simulink model "StaticVarCompensator"  (R2024a)
settings: Solver=FixedStepDiscrete  StartTime=0.0  StopTime=1  FixedStep=Ts  MaxStep=Ts*2  RelTol=1e-4  AbsTol=1e-4
PreLoadFcn:
  | Ts=50e-6;
undefined symbols (not defined in the file or in its folder): D1, Delta, DiscIntNeverNeededParam, find_system
libraries: spsSampleandHoldLib x24, spsThyristorLib x24, spsEdgeDetectorLib x12, spsSeriesRLCBranchLib x12, spsParallelRLCBranchLib x9, spsBistableLib x3, spsMeanVariableFrequencyLib x3, spsSecondOrderFilterLib x3, spsMultimeterLib x3, spsThreePhaseVIMeasurementLib x2, spsStairGeneratorLib x2, spsThreePhaseSeriesRLCLoadLib x1
(part 1 of 3)
settings Model: Creator=The MathWorks, Inc.  LastModifiedBy=Monia
settings SolverCC: AutoScaleAbsTol=off  AlgebraicLoopSolver=TrustRegion
settings DataIOCC: SaveFormat=StructureWithTime  SaveOutput=off  SignalLogging=off  DSMLogging=off  SaveTime=off  ReturnWorkspaceOutputs=off  SignalLoggingName=sigsOut
settings OptimizationCC: BooleanDataType=off  ExpressionDepthLimit=2147483647  InitFltsAndDblsToZero=on  EfficientMapNaN2IntZero=off  LifeSpan=inf
settings DebuggingCC: UnderspecifiedInitializationDetection=Classic  MergeDetectMultiDrivingBlocksExec=none  CheckExecutionContextPreStartOutputMsg=on  SignalResolutionControl=TryResolveAllWithWarning  MultiTaskDSMMsg=warning  MultiTaskCondExecSysMsg=none  FcnCallInpInsideContextMsg=warning  UnconnectedInputMsg=warning  UnconnectedOutputMsg=warning  UnconnectedLineMsg=warning  AllowSymbolicDim=off  StateNameClashWarn=warning  SFUnexpectedBacktrackingDiag=warning  SFNoUnconditionalDefaultTransitionDiag=warning  SFExecutionAtInitializationDiag=none  ArithmeticOperatorsInVariantConditions=warning
settings HardwareCC: ProdBitPerPointer=32  ProdBitPerSizeT=32  ProdBitPerPtrDiffT=32  ProdLargestAtomicFloat=None  ProdIntDivRoundTo=Undefined  ProdEndianess=Unspecified  ProdWordSize=32  ProdHWDeviceType=32-bit Generic  TargetUnknown=on
settings ModelReferenceCC: EnableRefExpFcnMdlSchedulingChecks=on  PropagateSignalLabelsOutOfModel=off
settings SFSimCC: SimUseLocalCustomCode=off  CustomCodeUndefinedFunction=UseInterfaceOnly
settings RTWCC: RTWUseLocalCustomCode=off  GPUComputeCapability=3.5  DLArmComputeVersion=19.05
settings CodeAppCC: StateflowObjectComments=on
settings GRTTargetCC: TargetLangStandard=C89/C90 (ANSI)  CombineOutputUpdateFcns=off  GRTInterface=on
settings ConfigComp: CovMetricSettings=dw  CovSaveCumulativeToWorkspaceVar=on  CovSaveSingleToWorkspaceVar=on  CovExternalEMLEnable=off  CovSFcnEnable=off
settings SimscapeCC: SimscapeNormalizeSystem=off

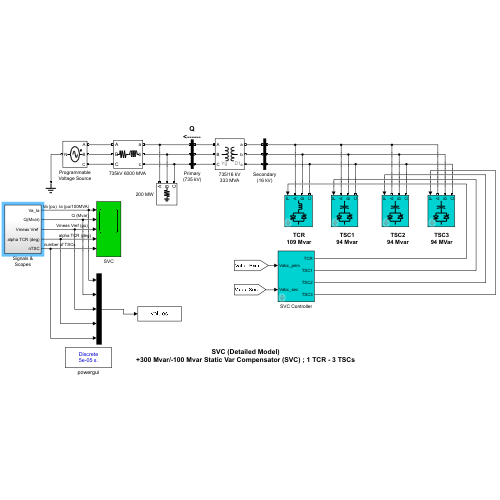
[thumbnail: Simulink's stored preview of the top-level diagram]
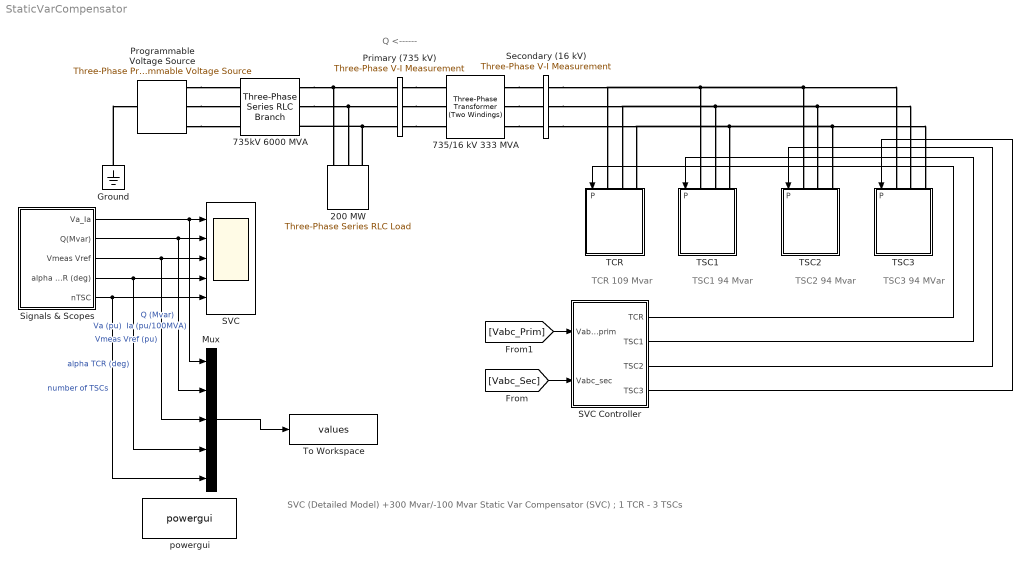
== system StaticVarCompensator ==
  note: SVC (Detailed Model)
      | +300 Mvar/-100 Mvar Static Var Compensator (SVC) ; 1 TCR - 3 TSCs
  note: TSC1
      | 94 Mvar
  note: TCR
      | 109 Mvar
  note: TSC2
      | 94 Mvar
  note: TSC3
      | 94 MVar
  note: Q
      | <------
  200 MW : spsThreePhaseSeriesRLCLoadLib/Three-Phase Series RLC Load  LConnTagsString=A|B|C  Configuration=Y (grounded)  NominalVoltage=735e3  Vabc=[1e3 1e3 1e3]  Vabcp=[1e3 1e3 1e3]  NominalFrequency=60  UnbalancedPower=off  ActivePower=200e6  InductivePower=0  CapacitivePower=0  Pabc=[10e3 9e3 11e3]  QLabc=[100 90 110]  QCabc=[100 90 110]  Pabcp=[10e3 9e3 11e3]  QLabcp=[100 90 110]  QCabcp=[100 90 110]  Measurements=None  LoadType=constant Z
  735/16 kV 333 MVA : spsThreePhaseTransformerTwoWindingsLib/Three-Phase Transformer (Two Windings)  Winding1Connection=Yg  Winding2Connection=Delta (D1)  CoreType=Three single-phase transformers  SetSaturation=off  Hysteresis=off  DataFile='hysteresis'  SetInitialFlux=off  Measurements=None  UNITS=pu  NominalPower=[333e6 , 60 ]  Winding1=[735e3 , 0.15/30/2 , 0.15*0.7]  Winding2=[ 16e3 , 0.15/30/2, 0.15*0.3]  Rm=500  Lm=500  L0=0.5  Saturation="[ 0,0  ;  0.005,1.2  ;  1.0,1.4 ]"  InitialFluxes=[ 0.8 , -0.8 , 0.7 ]  BreakLoop=off  DiscreteSolver=Trapezoidal iterative  DataType=off  TransfoNumber=0
  "735kV 6000 MVA " : spsThreePhaseSeriesRLCBranchLib/Three-Phase Series RLC Branch  LConnTagsString=A|B|C  RConnTagsString=A|B|C  BranchType=RL  Resistance=735e3^2/6000e6/10  Inductance=735e3^2/6000e6/(2*pi*60)  Capacitance=1.0  Measurements=None
  Ground : spsGroundLib/Ground  LConnTagsString=a
  Mux : Mux  Inputs=5
  Primary (735 kV) : spsThreePhaseVIMeasurementLib/Three-Phase V-I Measurement  VoltageMeasurement=phase-to-ground  SetLabelV=on  LabelV=Vabc_Prim  Vpu=on  VpuLL=off  CurrentMeasurement=yes  SetLabelI=on  LabelI=Iabc_Prim  Ipu=on  Pbase=100e6  Vbase=735e3  OutputType=Magnitude  PhasorSimulation=off  PSBequivalent=0
  Programmable Voltage Source : spsThreePhaseProgrammableVoltageSourceLib/Three-Phase Programmable Voltage Source  PositiveSequence="[1.004*735e3 0  60]"  VariationEntity=Amplitude  VariationType=Table of time-amplitude pairs  VariationTypeAlt=Step  VariationStep=-0.3  VariationRate=0.5  VariationMagnitude=0.4  VariationFrequency=2  VariationTiming=[0.1 1.2]  VariationPhaseA=off  Amplitudes=[1.0 1.025 0.93 1.0 ]  TimeValues=[0 0.1 0.4 0.7]  HarmonicGeneration=off  HarmonicA=[3 0.2 -25 0]  HarmonicB="[2 0.15  35 2]"  Timing="[0.1  0.6]"  BusType=swing  Pref=0  Qref=0  Qmin=-inf  Qmax=inf
  SVC : Scope  NumInputPorts=5
  SVC Controller : Subsystem  mask(SVC Controller){OpMode=Voltage regulation, Vref=1.0, KpKi=[0 800], Xs=0.01, Bmin_max=[-1.04  3.23], Bref=0, Ts=Ts}
      mask prompts: OpMode "Operation mode"; Vref "Reference voltage (pu):"; KpKi "Regulator gains [ Kp  Ki ]:"; Xs "Droop (pu/100MVA):"; Bmin_max "Min. and max. primary susceptances [ Bind Bcap] (pu/100MVA):"; Bref "Susceptance Bref (pu/100MVA) (Var control mode):"; Ts "Sample time (s):"
      mask help:
      | This block implements a controller for a Static Var Compensator (SVC) consisting of one thyristor-controlled reactor bank (TCR) and three thyristor-switched capacitor banks (TSCs). Outputs TCR, TSC1, TSC2 and TSC3 are vectors of six pulses for the TCR and the three TSCs.
      | In Voltage control mode the primary voltage (Vabc_prim) is controlled at Vref within the maximum inductive and capacitive susceptance range and droop setting. In Var control mode the SVC susceptance  is  kept constant at Bref (Bref<0 for inductive mode).
      | Thyristor pulses are synchronized on secondary line-to-line voltages (Vabc_sec) of the coupling transformer, assuming a Wye/Delta (D1) connection.
      mask init:
      | Kp=KpKi(1);
      | Ki=KpKi(2);
      | Bmin=Bmin_max(1);
      | Bmax=Bmin_max(2);
      mask TypeOptions OpMode: Voltage regulation | Var control (Fixed susceptance Bref)
  Secondary (16 kV) : spsThreePhaseVIMeasurementLib/Three-Phase V-I Measurement  VoltageMeasurement=phase-to-phase  SetLabelV=on  LabelV=Vabc_Sec  Vpu=on  VpuLL=off  CurrentMeasurement=no  SetLabelI=off  LabelI=Iabc_Sec  Ipu=off  Pbase=100e6  Vbase=16e3  OutputType=Magnitude  PhasorSimulation=off  PSBequivalent=0
  Signals & Scopes : Subsystem
  TCR : Subsystem  LoadFcn=find_system(gcs,'FollowLinks', 'on', 'LookUnderMasks', 'all');  mask(TCR branch){Ltcr=18.7e-3, Q=50, ParS=[500 250e-9], ParT=[1e-3  1*15]}
      mask prompts: Ltcr "TCR Inductance (H) :"; Q "Quality factor:"; ParS "Thyristor snubber: [ R (ohm)   C (F)  ]"; ParT "Thyristor data: [ Ron (ohm)   Vf (volt) ]"
      mask init:
      | Rtcr=(2*pi*60) * Ltcr / Q;
      | Rsnub=ParS(1);
      | Csnub=ParS(2);
      | Ron=ParT(1);
      | Vf=ParT(2);
      mask Display:
      | plot(0,0);plot(125,220)
      | plot([62 62 37 37 49 25 37],[15 39 39 58 76 76 58])
      | plot([62 87 87 99 87 75 87],[39 39 58 58 76 58 58])
      | plot([25 49],[58 58]);plot([37 25],[58 49])
      | plot([75 99],[76 76]);plot([87 99],[76 85])
      | plot([37 37 87 87],[76 95 95 76])
      | plot([62 62],[95 122]);plot([62 62],[164 186])
      | plot([62 72 78 79 78 72 62],[122 123 125 129 133 135 136])
      | plot([62 72 78 79 78 72 62],14+[122 123 125 129 133 135 136])
      | plot([62 72 78 79 78 72 62],28+[122 123 125 129 133 135 136])
  TSC1 : Subsystem  mask(TSC branch){Ccmt=308.4e-6, ParL=[1.13e-3 4.26e-3*2 191.7/2], ParS=[500 250e-9], ParT=[1e-3  1*15]}
      mask prompts: Ccmt "Capacitance (F) :"; ParL "[ Inductance (H)  Rseries (ohm)  Rparallel (ohm)  ]"; ParS "Thyristor snubber: [ R (ohm)   C (F)  ]"; ParT "Thyristor data: [ Ron (ohm)  Vf (volt) ]"
      mask init:
      | Lcmt=ParL(1);
      | Rseries=ParL(2);
      | Rparallel=ParL(3);
      | Rsnub=ParS(1);
      | Csnub=ParS(2);
      | Ron=ParT(1);
      | Vf=ParT(2);
      mask Display:
      | plot(0,0);plot(125,220)
      | plot([62 62 37 37 49 25 37],[15 39 39 58 76 76 58])
      | plot([62 87 87 99 87 75 87],[39 39 58 58 76 58 58])
      | plot([25 49],[58 58]);plot([37 25],[58 49])
      | plot([75 99],[76 76]);plot([87 99],[76 85])
      | plot([37 37 87 87],[76 95 95 76])
      | plot([62 62],[95 133]);plot([62 62],[164 183])
      | plot([62 69 73 78 81 82],13+[120 120 119 118 117 115])
      | plot([62 55 51 46 43 42],13+[120 120 119 118 117 115])
      | plot([42 82],[145 145])
      | plot([62 62],[145 164])
  TSC2 : Subsystem  mask(TSC branch){Ccmt=308.4e-6, ParL=[1.13e-3 4.26e-3*2 191.7/2], ParS=[500 250e-9], ParT=[1e-3 1*15]}
      mask prompts: Ccmt "Capacitance (F) :"; ParL "[ Inductance (H)  Rseries (ohm)  Rparallel (ohm)  ]"; ParS "Thyristor snubber: [ R (ohm)   C (F)  ]"; ParT "Thyristor data: [ Ron (ohm)  Vf (volt) ]"
      mask init:
      | Lcmt=ParL(1);
      | Rseries=ParL(2);
      | Rparallel=ParL(3);
      | Rsnub=ParS(1);
      | Csnub=ParS(2);
      | Ron=ParT(1);
      | Vf=ParT(2);
      mask Display:
      | plot(0,0);plot(125,220)
      | plot([62 62 37 37 49 25 37],[15 39 39 58 76 76 58])
      | plot([62 87 87 99 87 75 87],[39 39 58 58 76 58 58])
      | plot([25 49],[58 58]);plot([37 25],[58 49])
      | plot([75 99],[76 76]);plot([87 99],[76 85])
      | plot([37 37 87 87],[76 95 95 76])
      | plot([62 62],[95 133]);plot([62 62],[164 183])
      | plot([62 69 73 78 81 82],13+[120 120 119 118 117 115])
      | plot([62 55 51 46 43 42],13+[120 120 119 118 117 115])
      | plot([42 82],[145 145])
      | plot([62 62],[145 164])
  TSC3 : Subsystem  mask(TSC branch){Ccmt=308.4e-6, ParL=[1.13e-3 4.26e-3*2 191.7/2], ParS=[500 250e-9], ParT=[1e-3 1*15]}
      mask prompts: Ccmt "Capacitance (F) :"; ParL "[ Inductance (H)  Rseries (ohm)  Rparallel (ohm)  ]"; ParS "Thyristor snubber: [ R (ohm)   C (F)  ]"; ParT "Thyristor data: [ Ron (ohm)  Vf (volt) ]"
      mask init:
      | Lcmt=ParL(1);
      | Rseries=ParL(2);
      | Rparallel=ParL(3);
      | Rsnub=ParS(1);
      | Csnub=ParS(2);
      | Ron=ParT(1);
      | Vf=ParT(2);
      mask Display:
      | plot(0,0);plot(125,220)
      | plot([62 62 37 37 49 25 37],[15 39 39 58 76 76 58])
      | plot([62 87 87 99 87 75 87],[39 39 58 58 76 58 58])
      | plot([25 49],[58 58]);plot([37 25],[58 49])
      | plot([75 99],[76 76]);plot([87 99],[76 85])
      | plot([37 37 87 87],[76 95 95 76])
      | plot([62 62],[95 133]);plot([62 62],[164 183])
      | plot([62 69 73 78 81 82],13+[120 120 119 118 117 115])
      | plot([62 55 51 46 43 42],13+[120 120 119 118 117 115])
      | plot([42 82],[145 145])
      | plot([62 62],[145 164])
  To Workspace : ToWorkspace  VariableName=values  SaveFormat=Timeseries  SampleTime=-1
  powergui : spspowerguiLib/powergui  Priority=2  SimulationMode=Discrete  SampleTime=Ts  frequency=60  Iterations=50  frequencyindice=60  Pbase=100e6  ErrMax=1e-4  UnitsV=kV  UnitsW=MW  buscounter=0  FunctionMessages=off  echomessages=off  EnableUseOfTLC=off  CurrentSourceSwitches=off  DisableSnubberDevices=off  DisableRonSwitches=off  DisableVfSwitches=off  DisplayEquations=off  AutomaticDiscreteSolvers=off  SolverType=Tustin/Backward Euler (TBE)  Interpol=off  ExternalGateDelay=off  methode=off  Ts=0  x0status=blocks  SPID=off  SwTol=0  HookPort=off  NonlinearTolerance=0  nMaxIteration=15  ContinueOnMaxIteration=off  RestoreLinks=warning  ResistiveCurrentMeasurement=off  Frange=[0:2:500]  Ylog=off  Xlog=on  ShowGrid=off  save=off  variable=ZData  structure=0  ZoomFFT=on  StartTime=0.0  cycles=1  DisplayStyle=1  fundamental=60  FreqAxis=off  MaxFrequency=1000  frequencyindicesteady=1  RmsSteady=2  display=off
  wires:
  [Vabc_Sec] -> SVC Controller/2(Vabc_sec)
  [Vabc_Prim] -> SVC Controller/1(Vabc_prim)
  Signals & Scopes/1(Va_Ia) -> Mux/1, SVC/1  "Va (pu)  Ia (pu/100MVA)"
  SVC Controller/1(TCR) -> TCR/1(P)
  SVC Controller/2(TSC1) -> TSC1/1(P)
  SVC Controller/3(TSC2) -> TSC2/1(P)
  SVC Controller/4(TSC3) -> TSC3/1(P)
  Signals & Scopes/3("Vmeas Vref ") -> Mux/3, SVC/3  "Vmeas Vref (pu)"
  Signals & Scopes/5(nTSC) -> Mux/5, SVC/5  "number of TSCs"
  Signals & Scopes/2(Q(Mvar)) -> Mux/2, SVC/2  "Q (Mvar)"
  Signals & Scopes/4(alpha TCR (deg)) -> Mux/4, SVC/4  "alpha TCR (deg)"
  Mux/1 -> To Workspace/1
  connections:
  Ground/LConn1 -- Programmable Voltage Source/LConn1
  "735kV 6000 MVA "/RConn1 -- Primary (735 kV)/LConn1 -- 200 MW/LConn1
  "735kV 6000 MVA "/RConn2 -- Primary (735 kV)/LConn2 -- 200 MW/LConn2
  735/16 kV 333 MVA/RConn1 -- Secondary (16 kV)/LConn1
  735/16 kV 333 MVA/RConn3 -- Secondary (16 kV)/LConn3
  Programmable Voltage Source/RConn2 -- "735kV 6000 MVA "/LConn2
  Programmable Voltage Source/RConn3 -- "735kV 6000 MVA "/LConn3
  Programmable Voltage Source/RConn1 -- "735kV 6000 MVA "/LConn1
  735/16 kV 333 MVA/RConn2 -- Secondary (16 kV)/LConn2
  200 MW/LConn3 -- Primary (735 kV)/LConn3 -- "735kV 6000 MVA "/RConn3
  Secondary (16 kV)/RConn1 -- TCR/LConn1 -- TSC1/LConn1 -- TSC2/LConn1 -- TSC3/LConn1
  Secondary (16 kV)/RConn2 -- TCR/LConn2 -- TSC1/LConn2 -- TSC2/LConn2 -- TSC3/LConn2
  Secondary (16 kV)/RConn3 -- TCR/LConn3 -- TSC1/LConn3 -- TSC2/LConn3 -- TSC3/LConn3
  Primary (735 kV)/RConn1 -- 735/16 kV 333 MVA/LConn1
  Primary (735 kV)/RConn2 -- 735/16 kV 333 MVA/LConn2
  Primary (735 kV)/RConn3 -- 735/16 kV 333 MVA/LConn3

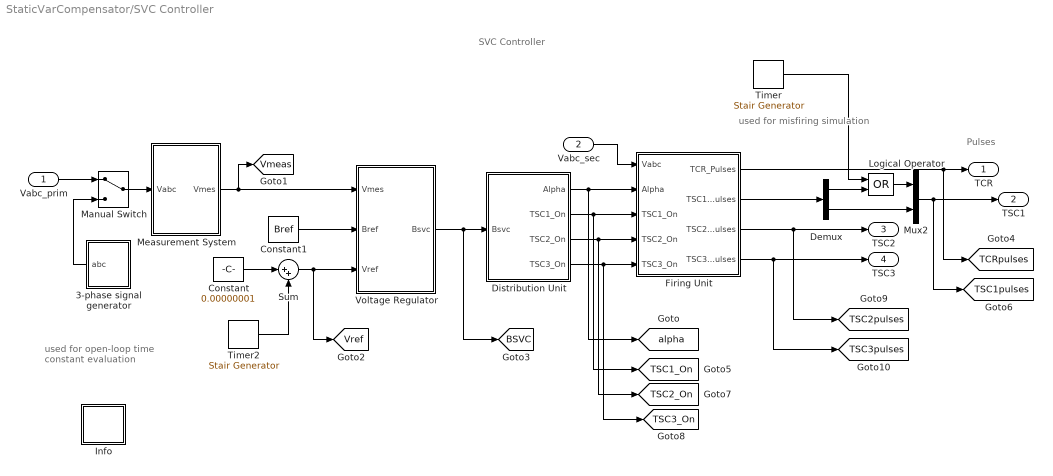
== system StaticVarCompensator/SVC Controller ==
  note: Pulses
  note: SVC Controller
  note: used for misfiring
      | simulation
  note: used for open-loop
      | time constant evaluation
  Vabc_prim : Inport  PortDimensions=3
  Vabc_sec : Inport  Port=2  PortDimensions=3
  3-phase signal generator : Subsystem
  Constant : Constant  Value=0.00000001
  Constant1 : Constant  Value=Bref
  Demux : Demux  Outputs=[1 5]
      settings: DisplayOption=none
  Distribution Unit : Subsystem  mask(Distribution Unit){ParNom=[333e6 60], Xf_xfo=0.15, Vsec_svc=16e3, L_TCR=18.7e-3, C_TSC=308.4e-6, L_TSC=1.13e-3, hyst_svc=0.1, Ts=Ts}
      mask prompts: ParNom "Transformer nominal power and frequency: [  P (VA)    Freq (Hz)  ]"; Xf_xfo "Transformer total leakage (pu/Pnom):"; Vsec_svc "Nominal secondary voltage (Volts rms ph-ph):"; L_TCR "TCR branch inductance (H):"; C_TSC "TSC branch capacitance (F):"; L_TSC "TSC branch inductance (H)"; hyst_svc "Hysteresis - Distribution unit (pu/100MVA):"; Ts "Sample time:"
      mask init:
      | Pnom_xfo=ParNom(1);
      | Freq=ParNom(2);
      | Bsec_pu100=100e6/Vsec_svc/Vsec_svc/3;
      | w=2*pi*Freq;
      | Bpu_TCR=-1/L_TCR/w/Bsec_pu100;
      | Bpu_TSC=1/(1/w/C_TSC-L_TSC*w)/Bsec_pu100;
      | B=1:-0.0025:0.0;
      | B=B';
      | for i=1:401,
      |       if B(i) <= 0,
      | 	ang = 0;
      |       elseif B(i) >= 1,
      | 	ang = pi;
      |       else,
      | 	a = pi; e = .0001;
      | 	da = a;
      | 	while abs(da)>e,
      | 		da = (pi*B(i)-a+sin(a))/(1-cos(a));
      | 		a = a + da;
      | 	end;
      | 	ang = a;
      |       end;
      |       A(i)=(180-ang*180/pi)/2+90;
      | end
      | A=A';
      | B=-B;
  Firing Unit : Subsystem  mask(Firing Unit){FiringMode=Synchronized, Nstep=0, ParInit=[0 60], Ts=Ts}
      mask prompts: FiringMode "Firing mode"; Nstep "Total delay (in number of time step)"; ParInit "Initial phase and frequency of input: [ Phase (degree)  Freq (Hz) ]"; Ts "Sample time:"
      mask init:
      | PhaseInit=ParInit(1);
      | FreqInit=ParInit(2);
      mask TypeOptions FiringMode: Synchronized | Continuous
  Info : Subsystem
      mask Display: disp('?')
  Logical Operator : Logic  Operator=OR
  Manual Switch : ManualSwitch
  Measurement System : Subsystem  mask(SVC measurement system){Vnom=735e3, ParI=[735e3*0.9998 0 60], Ts=Ts}
      mask prompts: Vnom "Nominal voltage (volts rms ph-ph)"; ParI "Initial input: [ Mag (volts rms ph-ph)  Phase (degree) Freq (Hz) ]"; Ts "Sample time:"
      mask init:
      | Mag_Init=ParI(1)/Vnom;
      | Phase_Init=ParI(2);
      | Freq_Init=ParI(3);
  Mux2 : Mux  Inputs=[1 5]
  Sum : Sum  Inputs=|++  SaturateOnIntegerOverflow=on
  Timer : spsStairGeneratorLib/Stair Generator  t="[ 0  0.121  0.121+eps ]*100"  e="[0  1  0 ]"  Ts=Ts
  Timer2 : spsStairGeneratorLib/Stair Generator  t="[ 0  0.4  0.6 ]"  e=[1 1 1 ]  Ts=Ts
  Voltage Regulator : Subsystem
  TCR : Outport  VectorParamsAs1DForOutWhenUnconnected=off
  TSC1 : Outport  Port=2  VectorParamsAs1DForOutWhenUnconnected=off
  TSC2 : Outport  Port=3  VectorParamsAs1DForOutWhenUnconnected=off
  TSC3 : Outport  Port=4  VectorParamsAs1DForOutWhenUnconnected=off
  tag scope: BSVC=global, TCRpulses=global, TSC1_On=global, TSC1pulses=global, TSC2_On=global, TSC2pulses=global, TSC3_On=global, TSC3pulses=global, Vmeas=global, Vref=global, alpha=global
  wires:
  Timer/1 -> Logical Operator/1
  Firing Unit/2(TSC1_Pulses) -> Demux/1
  Measurement System/1(Vmes) -> Voltage Regulator/1(Vmes), [Vmeas]
  Constant1/1 -> Voltage Regulator/2(Bref)
  Mux2/1 -> TSC1/1, [TSC1pulses]
  Demux/2 -> Mux2/2
  Logical Operator/1 -> Mux2/1
  Demux/1 -> Logical Operator/2
  Voltage Regulator/1(Bsvc) -> Distribution Unit/1(Bsvc), [BSVC]
  Sum/1 -> [Vref], Voltage Regulator/3(Vref)
  Constant/1 -> Sum/1
  Vabc_prim/1 -> Manual Switch/1
  Manual Switch/1 -> Measurement System/1(Vabc)
  3-phase signal generator/1(abc) -> Manual Switch/2
  Firing Unit/1(TCR_Pulses) -> TCR/1, [TCRpulses]
  Firing Unit/3(TSC2_Pulses) -> TSC2/1, [TSC2pulses]
  Firing Unit/4(TSC3_Pulses) -> TSC3/1, [TSC3pulses]
  Distribution Unit/1(Alpha) -> Firing Unit/2(Alpha), [alpha]
  Distribution Unit/2(TSC1_On) -> Firing Unit/3(TSC1_On), [TSC1_On]
  Distribution Unit/3(TSC2_On) -> Firing Unit/4(TSC2_On), [TSC2_On]
  Distribution Unit/4(TSC3_On) -> Firing Unit/5(TSC3_On), [TSC3_On]
  Vabc_sec/1 -> Firing Unit/1(Vabc)
  Timer2/1 -> Sum/2

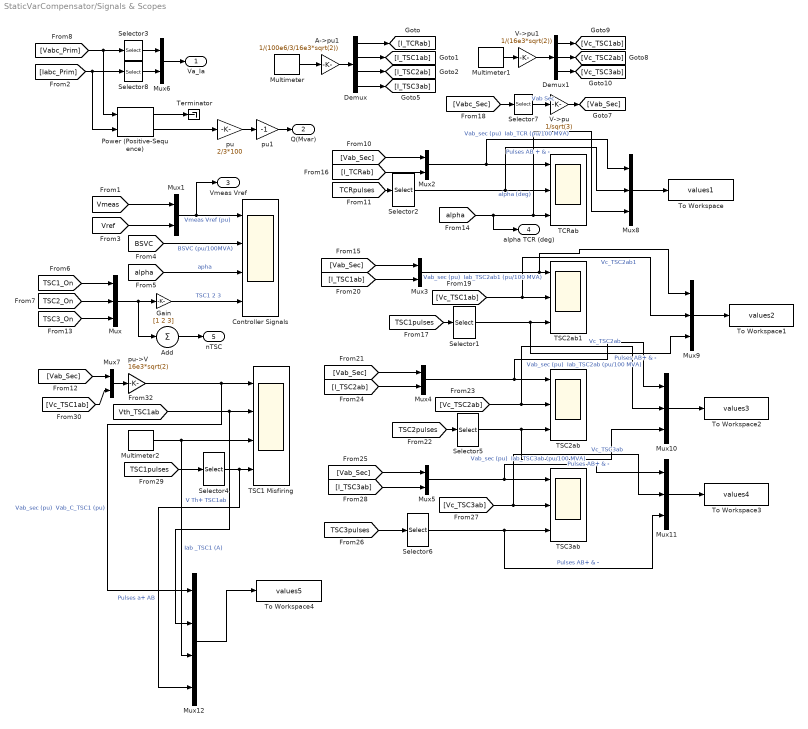
== system StaticVarCompensator/Signals & Scopes ==
  A->pu1 : Gain  Gain=1/(100e6/3/16e3*sqrt(2))  SaturateOnIntegerOverflow=on  OutDataTypeStr=Inherit: Same as input  ParamDataTypeStr=Inherit: Same as input
  Add : Sum  Inputs=+
  Controller Signals : Scope  NumInputPorts=4
  Demux : Demux
      settings: DisplayOption=none
  Demux1 : Demux  Outputs=3
      settings: DisplayOption=none
  Gain : Gain  Gain=[1 2 3]  SaturateOnIntegerOverflow=on  OutDataTypeStr=Inherit: Same as input  ParamDataTypeStr=Inherit: Same as input
  Multimeter : spsMultimeterLib/Multimeter  Tag=PoWeRsYsTeMmEaSuReMeNt  L=7  sel=[4 5 6 7]  yselected={}  Gain=[1 1 1 1]  OutputType=Magnitude  PlotAtSimulationStop=off  PhasorSimulation=off
      settings: AttributesFormatString=\n
  Multimeter1 : spsMultimeterLib/Multimeter  Tag=PoWeRsYsTeMmEaSuReMeNt  L=7  sel=[1 2 3]  yselected={}  Gain=[1 1 1]  OutputType=Magnitude  PlotAtSimulationStop=off  PhasorSimulation=off
      settings: AttributesFormatString=\n
  Multimeter2 : spsMultimeterLib/Multimeter  Tag=PoWeRsYsTeMmEaSuReMeNt  L=7  sel=5  yselected={}  Gain=1  OutputType=Magnitude  PlotAtSimulationStop=off  PhasorSimulation=off
      settings: AttributesFormatString=\n
  Mux{,8..11} (5 alike) : Mux  Inputs=3
  Mux{1..7} (7 alike) : Mux  Inputs=2
  Mux12 : Mux
  Power (Positive-Sequence) : spsPowerPositiveSequenceLib/Power (Positive-Sequence)  Freq=60  Vinit=[1 0]  Iinit=[0.05 90]  Ts=Ts
  Selector{1..2,5..6} (4 alike) : Selector  InputPortWidth=6  IndexOptions=Index vector (dialog)  Indices=[1 2]  OutputSizes=1
  Selector3 : Selector  InputPortWidth=3  IndexOptions=Index vector (dialog)  Indices=1  OutputSizes=1
  Selector4 : Selector  InputPortWidth=6  IndexOptions=Index vector (dialog)  Indices=[1 ]  OutputSizes=1
  Selector7 : Selector  InputPortWidth=3  IndexOptions=Index vector (dialog)  Indices=1  OutputSizes=1
  Selector8 : Selector  InputPortWidth=3  IndexOptions=Index vector (dialog)  Indices=1  OutputSizes=1
  TCRab : Scope  NumInputPorts=3
  TSC1 Misfiring : Scope  NumInputPorts=4
  TSC2ab : Scope  NumInputPorts=3
  TSC2ab1 : Scope  NumInputPorts=3
  TSC3ab : Scope  NumInputPorts=3
  Terminator : Terminator
  To Workspace : ToWorkspace  VariableName=values1  SaveFormat=Timeseries  SampleTime=-1
  To Workspace1 : ToWorkspace  VariableName=values2  SaveFormat=Timeseries  SampleTime=-1
  To Workspace2 : ToWorkspace  VariableName=values3  SaveFormat=Timeseries  SampleTime=-1
  To Workspace3 : ToWorkspace  VariableName=values4  SaveFormat=Timeseries  SampleTime=-1
  To Workspace4 : ToWorkspace  VariableName=values5  SaveFormat=Timeseries  SampleTime=-1
  "V->pu " : Gain  Gain=1/sqrt(3)  SaturateOnIntegerOverflow=on  OutDataTypeStr=Inherit: Same as input  ParamDataTypeStr=Inherit: Same as input
  V->pu1 : Gain  Gain=1/(16e3*sqrt(2))  SaturateOnIntegerOverflow=on  OutDataTypeStr=Inherit: Same as input  ParamDataTypeStr=Inherit: Same as input
  pu : Gain  Gain=2/3*100  SaturateOnIntegerOverflow=on  OutDataTypeStr=Inherit: Same as input  ParamDataTypeStr=Inherit: Same as input
  pu->V : Gain  Gain=16e3*sqrt(2)  SaturateOnIntegerOverflow=on  OutDataTypeStr=Inherit: Same as input  ParamDataTypeStr=Inherit: Same as input
  pu1 : Gain  Gain=-1  SaturateOnIntegerOverflow=on  OutDataTypeStr=Inherit: Same as input  ParamDataTypeStr=Inherit: Same as input
  Va_Ia : Outport  VectorParamsAs1DForOutWhenUnconnected=off
  Q(Mvar) : Outport  Port=2  VectorParamsAs1DForOutWhenUnconnected=off
  "Vmeas Vref " : Outport  Port=3  VectorParamsAs1DForOutWhenUnconnected=off
  alpha TCR (deg) : Outport  Port=4  VectorParamsAs1DForOutWhenUnconnected=off
  nTSC : Outport  Port=5  VectorParamsAs1DForOutWhenUnconnected=off
  wires:
  [TSC1_On] -> Mux/1
  [TSC2_On] -> Mux/2
  Mux/1 -> Gain/1, Add/1
  [Vmeas] -> Mux1/1
  [Vref] -> Mux1/2
  [Vabc_Prim] -> Power (Positive-Sequence)/1, Selector3/1
  [Iabc_Prim] -> Power (Positive-Sequence)/2, Selector8/1
  Power (Positive-Sequence)/1 -> Terminator/1
  pu/1 -> pu1/1
  [BSVC] -> Controller Signals/2  "BSVC (pu/100MVA)"
  Mux1/1 -> Controller Signals/1, "Vmeas Vref "/1  "Vmeas Vref (pu)"
  [alpha] -> Controller Signals/3  "apha"
  Gain/1 -> Controller Signals/4  "TSC1 2 3"
  [TSC3_On] -> Mux/3
  Multimeter/1 -> A->pu1/1
  [TCRpulses] -> Selector2/1
  Selector2/1 -> Mux8/2, TCRab/2  "Pulses AB + & -"
  Demux/1 -> [I_TCRab]
  Demux/4 -> [I_TSC3ab]
  [Vabc_Sec] -> Selector7/1
  Selector7/1 -> "V->pu "/1  "Vab Sec"
  [alpha] -> Mux8/3, TCRab/3, alpha TCR (deg)/1  "alpha (deg)"
  [Vab_Sec] -> Mux2/1
  [I_TCRab] -> Mux2/2
  Mux2/1 -> Mux8/1, TCRab/1  "Vab_sec (pu)  Iab_TCR (pu/100 MVA)"
  [Vab_Sec] -> Mux3/1
  [I_TSC1ab] -> Mux3/2
  [TSC1pulses] -> Selector1/1
  "V->pu "/1 -> [Vab_Sec]
  Demux/2 -> [I_TSC1ab]
  Demux/3 -> [I_TSC2ab]
  Multimeter1/1 -> V->pu1/1
  Demux1/1 -> [Vc_TSC1ab]
  Demux1/2 -> [Vc_TSC2ab]
  Demux1/3 -> [Vc_TSC3ab]
  [Vab_Sec] -> Mux4/1
  [I_TSC2ab] -> Mux4/2
  [TSC2pulses] -> Selector5/1
  [Vab_Sec] -> Mux5/1
  [I_TSC3ab] -> Mux5/2
  [TSC3pulses] -> Selector6/1
  pu1/1 -> Q(Mvar)/1
  Add/1 -> nTSC/1
  Selector3/1 -> Mux6/1
  Selector8/1 -> Mux6/2
  Mux6/1 -> Va_Ia/1
  [Vab_Sec] -> Mux7/1
  Mux7/1 -> pu->V/1
  [TSC1pulses] -> Selector4/1
  Selector4/1 -> Mux12/4, TSC1 Misfiring/4  "Pulses a+ AB"
  A->pu1/1 -> Demux/1
  V->pu1/1 -> Demux1/1
  [Vc_TSC1ab] -> Mux7/2
  Multimeter2/1 -> TSC1 Misfiring/3, Mux12/3  "Iab _TSC1 (A)"
  [Vth_TSC1ab] -> Mux12/2, TSC1 Misfiring/2  "V Th+ TSC1ab"
  pu->V/1 -> Mux12/1, TSC1 Misfiring/1  "Vab_sec (pu)  Vab_C_TSC1 (pu)"
  Power (Positive-Sequence)/2 -> pu/1
  Mux8/1 -> To Workspace/1
  Mux9/1 -> To Workspace1/1
  [Vc_TSC1ab] -> Mux9/2, TSC2ab1/2  "Vc_TSC2ab1"
  Mux3/1 -> Mux9/1, TSC2ab1/1  "Vab_sec (pu)  Iab_TSC2ab1 (pu/100 MVA)"
  Selector1/1 -> Mux9/3, TSC2ab1/3  "Pulses AB+ & -"
  Mux10/1 -> To Workspace2/1
  Mux4/1 -> Mux10/1, TSC2ab/1  "Vab_sec (pu)  Iab_TSC2ab (pu/100 MVA)"
  Selector5/1 -> Mux10/3, TSC2ab/3  "Pulses AB+ & -"
  [Vc_TSC2ab] -> Mux10/2, TSC2ab/2  "Vc_TSC2ab"
  Mux11/1 -> To Workspace3/1
  Mux5/1 -> Mux11/1, TSC3ab/1  "Vab_sec (pu)  Iab_TSC3ab (pu/100 MVA)"
  [Vc_TSC3ab] -> Mux11/2, TSC3ab/2  "Vc_TSC3ab"
  Selector6/1 -> Mux11/3, TSC3ab/3  "Pulses AB+ & -"
  Mux12/1 -> To Workspace4/1

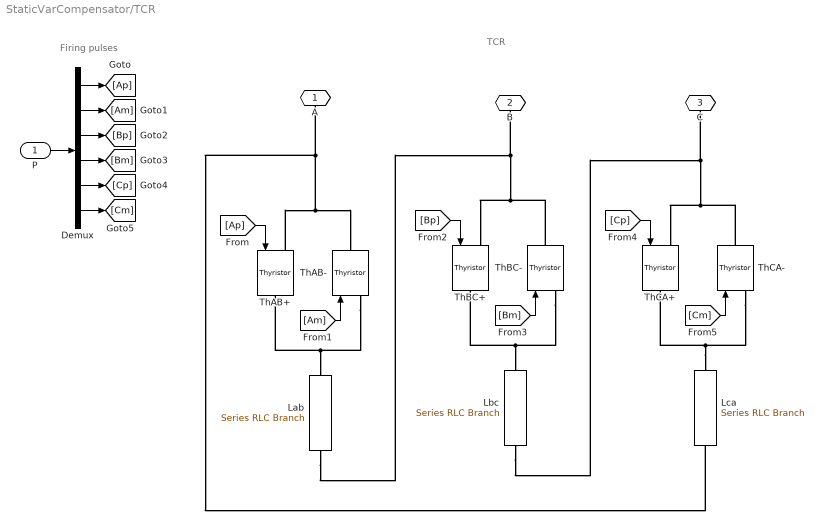
== system StaticVarCompensator/TCR ==
  note: Firing pulses
  note: TCR
  P : Inport  PortDimensions=6
  Demux : Demux  Outputs=6
      settings: DisplayOption=none
  Lab : spsSeriesRLCBranchLib/Series RLC Branch  LConnTagsString=__new0  RConnTagsString=__new0  BranchType=RL  Resistance=Rtcr  Inductance=Ltcr  SetiL0=off  InitialCurrent=0  Capacitance=1.0  Setx0=off  InitialVoltage=0  Measurements=Branch current
  Lbc : spsSeriesRLCBranchLib/Series RLC Branch  LConnTagsString=__new0  RConnTagsString=__new0  BranchType=RL  Resistance=Rtcr  Inductance=Ltcr  SetiL0=off  InitialCurrent=0  Capacitance=1.0  Setx0=off  InitialVoltage=0  Measurements=None
  Lca : spsSeriesRLCBranchLib/Series RLC Branch  LConnTagsString=__new0  RConnTagsString=__new0  BranchType=RL  Resistance=Rtcr  Inductance=Ltcr  SetiL0=off  InitialCurrent=0  Capacitance=1.0  Setx0=off  InitialVoltage=0  Measurements=None
  ThAB+ : spsThyristorLib/Thyristor  Ron=Ron  Lon=0  Vf=Vf  IC=0  Rs=Rsnub  Cs=Csnub  Measurements=off
      settings: AttributesFormatString=\n
  ThAB- : spsThyristorLib/Thyristor  Ron=Ron  Lon=0  Vf=Vf  IC=0  Rs=inf  Cs=0  Measurements=off
      settings: AttributesFormatString=\n
  ThBC+ : spsThyristorLib/Thyristor  Ron=Ron  Lon=0  Vf=Vf  IC=0  Rs=Rsnub  Cs=Csnub  Measurements=off
      settings: AttributesFormatString=\n
  ThBC- : spsThyristorLib/Thyristor  Ron=Ron  Lon=0  Vf=Vf  IC=0  Rs=inf  Cs=0  Measurements=off
      settings: AttributesFormatString=\n
  ThCA+ : spsThyristorLib/Thyristor  Ron=Ron  Lon=0  Vf=Vf  IC=0  Rs=Rsnub  Cs=Csnub  Measurements=off
      settings: AttributesFormatString=\n
  ThCA- : spsThyristorLib/Thyristor  Ron=Ron  Lon=0  Vf=Vf  IC=0  Rs=inf  Cs=0  Measurements=off
      settings: AttributesFormatString=\n
  A : PMIOPort  Side=Left
  B : PMIOPort  Port=2  Side=Left
  C : PMIOPort  Port=3  Side=Left
  wires:
  P/1 -> Demux/1
  Demux/1 -> [Ap]
  Demux/2 -> [Am]
  Demux/3 -> [Bp]
  Demux/4 -> [Bm]
  Demux/5 -> [Cp]
  [Cp] -> ThCA+/1
  [Cm] -> ThCA-/1
  Demux/6 -> [Cm]
  [Bm] -> ThBC-/1
  [Bp] -> ThBC+/1
  [Am] -> ThAB-/1
  [Ap] -> ThAB+/1
  connections:
  ThAB-/LConn1 -- ThAB+/RConn1 -- Lab/LConn1
  ThAB+/LConn1 -- ThAB-/RConn1 -- Lca/RConn1 -- A/RConn1
  ThBC-/LConn1 -- Lbc/LConn1 -- ThBC+/RConn1
  Lab/RConn1 -- ThBC-/RConn1 -- ThBC+/LConn1 -- B/RConn1
  Lca/LConn1 -- ThCA-/LConn1 -- ThCA+/RConn1
  Lbc/RConn1 -- ThCA-/RConn1 -- ThCA+/LConn1 -- C/RConn1

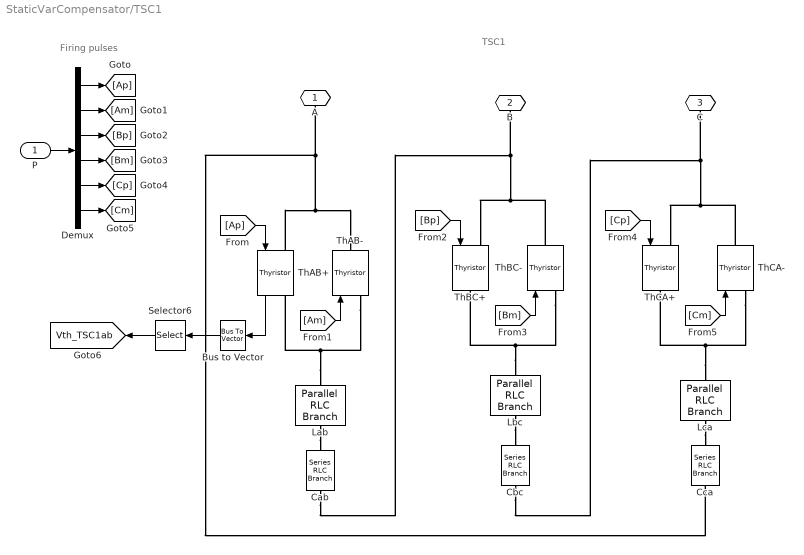
== system StaticVarCompensator/TSC1 ==
  note: Firing pulses
  note: TSC1
  P : Inport  PortDimensions=6
  Bus to Vector : BusToVector
  Cab : spsSeriesRLCBranchLib/Series RLC Branch  LConnTagsString=__new0  RConnTagsString=__new0  BranchType=RC  Resistance=Rseries  Inductance=1.0  SetiL0=off  InitialCurrent=0  Capacitance=Ccmt  Setx0=off  InitialVoltage=0  Measurements=Branch voltage and current
  Cbc : spsSeriesRLCBranchLib/Series RLC Branch  LConnTagsString=__new0  RConnTagsString=__new0  BranchType=RC  Resistance=Rseries  Inductance=1.0  SetiL0=off  InitialCurrent=0  Capacitance=Ccmt  Setx0=off  InitialVoltage=0  Measurements=None
  Cca : spsSeriesRLCBranchLib/Series RLC Branch  LConnTagsString=__new0  RConnTagsString=__new0  BranchType=RC  Resistance=Rseries  Inductance=1.0  SetiL0=off  InitialCurrent=0  Capacitance=Ccmt  Setx0=off  InitialVoltage=0  Measurements=None
  Demux : Demux  Outputs=6
      settings: DisplayOption=none
  Lab : spsParallelRLCBranchLib/Parallel RLC Branch  LConnTagsString=a  RConnTagsString=__new0  BranchType=RL  Resistance=Rparallel  Inductance=Lcmt  SetiL0=off  InitialCurrent=0  Capacitance=1.0  Setx0=off  InitialVoltage=0  Measurements=None
  Lbc : spsParallelRLCBranchLib/Parallel RLC Branch  LConnTagsString=a  RConnTagsString=__new0  BranchType=RL  Resistance=Rparallel  Inductance=Lcmt  SetiL0=off  InitialCurrent=0  Capacitance=1.0  Setx0=off  InitialVoltage=0  Measurements=None
  Lca : spsParallelRLCBranchLib/Parallel RLC Branch  LConnTagsString=a  RConnTagsString=__new0  BranchType=RL  Resistance=Rparallel  Inductance=Lcmt  SetiL0=off  InitialCurrent=0  Capacitance=1.0  Setx0=off  InitialVoltage=0  Measurements=None
  Selector6 : Selector  InputPortWidth=2  IndexOptions=Index vector (dialog)  Indices=2  OutputSizes=1
  ThAB+ : spsThyristorLib/Thyristor  Ron=Ron  Lon=0  Vf=Vf  IC=0  Rs=Rsnub  Cs=Csnub  Measurements=on
      settings: AttributesFormatString=\n
  ThAB- : spsThyristorLib/Thyristor  Ron=Ron  Lon=0  Vf=Vf  IC=0  Rs=inf  Cs=0  Measurements=off
      settings: AttributesFormatString=\n
  ThBC+ : spsThyristorLib/Thyristor  Ron=Ron  Lon=0  Vf=Vf  IC=0  Rs=Rsnub  Cs=Csnub  Measurements=off
      settings: AttributesFormatString=\n
  ThBC- : spsThyristorLib/Thyristor  Ron=Ron  Lon=0  Vf=Vf  IC=0  Rs=inf  Cs=0  Measurements=off
      settings: AttributesFormatString=\n
  ThCA+ : spsThyristorLib/Thyristor  Ron=Ron  Lon=0  Vf=Vf  IC=0  Rs=Rsnub  Cs=Csnub  Measurements=off
      settings: AttributesFormatString=\n
  ThCA- : spsThyristorLib/Thyristor  Ron=Ron  Lon=0  Vf=Vf  IC=0  Rs=inf  Cs=0  Measurements=off
      settings: AttributesFormatString=\n
  A : PMIOPort  Side=Left
  B : PMIOPort  Port=2  Side=Left
  C : PMIOPort  Port=3  Side=Left
  tag scope: Vth_TSC1ab=global
  wires:
  P/1 -> Demux/1
  [Ap] -> ThAB+/1
  Demux/1 -> [Ap]
  Demux/2 -> [Am]
  Demux/3 -> [Bp]
  Demux/4 -> [Bm]
  Demux/5 -> [Cp]
  [Am] -> ThAB-/1
  [Bp] -> ThBC+/1
  [Bm] -> ThBC-/1
  [Cp] -> ThCA+/1
  [Cm] -> ThCA-/1
  Demux/6 -> [Cm]
  ThAB+/1 -> Bus to Vector/1
  Selector6/1 -> [Vth_TSC1ab]
  Bus to Vector/1 -> Selector6/1
  connections:
  Lab/RConn1 -- Cab/LConn1
  Lab/LConn1 -- ThAB-/LConn1 -- ThAB+/RConn1
  Cca/RConn1 -- A/RConn1 -- ThAB+/LConn1 -- ThAB-/RConn1
  Lbc/LConn1 -- ThBC-/LConn1 -- ThBC+/RConn1
  Cab/RConn1 -- ThBC-/RConn1 -- ThBC+/LConn1 -- B/RConn1
  Lca/LConn1 -- ThCA-/LConn1 -- ThCA+/RConn1
  Cbc/RConn1 -- ThCA-/RConn1 -- ThCA+/LConn1 -- C/RConn1
  Lbc/RConn1 -- Cbc/LConn1
  Lca/RConn1 -- Cca/LConn1

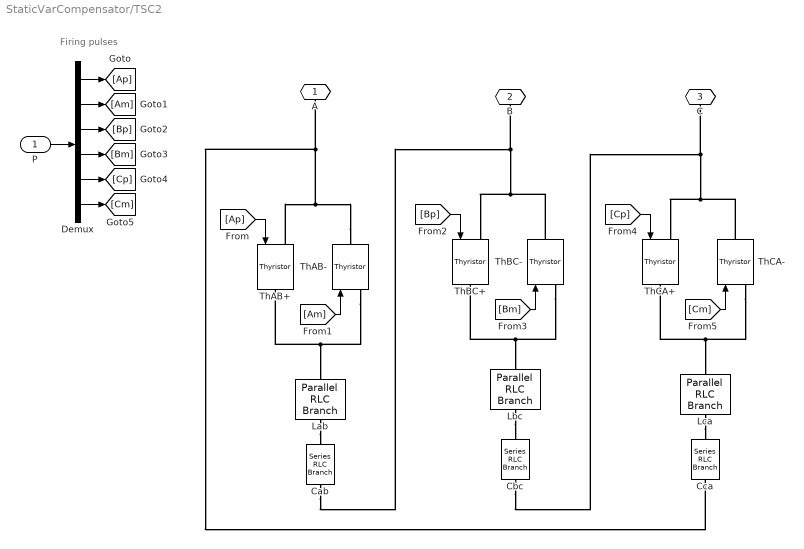
== system StaticVarCompensator/TSC2 ==
  note: Firing pulses
  P : Inport  PortDimensions=6
  Cab : spsSeriesRLCBranchLib/Series RLC Branch  LConnTagsString=__new0  RConnTagsString=__new0  BranchType=RC  Resistance=Rseries  Inductance=1.0  SetiL0=off  InitialCurrent=0  Capacitance=Ccmt  Setx0=off  InitialVoltage=0  Measurements=Branch voltage and current
  Cbc : spsSeriesRLCBranchLib/Series RLC Branch  LConnTagsString=__new0  RConnTagsString=__new0  BranchType=RC  Resistance=Rseries  Inductance=1.0  SetiL0=off  InitialCurrent=0  Capacitance=Ccmt  Setx0=off  InitialVoltage=0  Measurements=None
  Cca : spsSeriesRLCBranchLib/Series RLC Branch  LConnTagsString=__new0  RConnTagsString=__new0  BranchType=RC  Resistance=Rseries  Inductance=1.0  SetiL0=off  InitialCurrent=0  Capacitance=Ccmt  Setx0=off  InitialVoltage=0  Measurements=None
  Demux : Demux  Outputs=6
      settings: DisplayOption=none
  Lab : spsParallelRLCBranchLib/Parallel RLC Branch  LConnTagsString=a  RConnTagsString=__new0  BranchType=RL  Resistance=Rparallel  Inductance=Lcmt  SetiL0=off  InitialCurrent=0  Capacitance=1.0  Setx0=off  InitialVoltage=0  Measurements=None
  Lbc : spsParallelRLCBranchLib/Parallel RLC Branch  LConnTagsString=a  RConnTagsString=__new0  BranchType=RL  Resistance=Rparallel  Inductance=Lcmt  SetiL0=off  InitialCurrent=0  Capacitance=1.0  Setx0=off  InitialVoltage=0  Measurements=None
  Lca : spsParallelRLCBranchLib/Parallel RLC Branch  LConnTagsString=a  RConnTagsString=__new0  BranchType=RL  Resistance=Rparallel  Inductance=Lcmt  SetiL0=off  InitialCurrent=0  Capacitance=1.0  Setx0=off  InitialVoltage=0  Measurements=None
  ThAB+ : spsThyristorLib/Thyristor  Ron=Ron  Lon=0  Vf=Vf  IC=0  Rs=Rsnub  Cs=Csnub  Measurements=off
      settings: AttributesFormatString=\n
  ThAB- : spsThyristorLib/Thyristor  Ron=Ron  Lon=0  Vf=Vf  IC=0  Rs=inf  Cs=0  Measurements=off
      settings: AttributesFormatString=\n
  ThBC+ : spsThyristorLib/Thyristor  Ron=Ron  Lon=0  Vf=Vf  IC=0  Rs=Rsnub  Cs=Csnub  Measurements=off
      settings: AttributesFormatString=\n
  ThBC- : spsThyristorLib/Thyristor  Ron=Ron  Lon=0  Vf=Vf  IC=0  Rs=inf  Cs=0  Measurements=off
      settings: AttributesFormatString=\n
  ThCA+ : spsThyristorLib/Thyristor  Ron=Ron  Lon=0  Vf=Vf  IC=0  Rs=Rsnub  Cs=Csnub  Measurements=off
      settings: AttributesFormatString=\n
  ThCA- : spsThyristorLib/Thyristor  Ron=Ron  Lon=0  Vf=Vf  IC=0  Rs=inf  Cs=0  Measurements=off
      settings: AttributesFormatString=\n
  A : PMIOPort  Side=Left
  B : PMIOPort  Port=2  Side=Left
  C : PMIOPort  Port=3  Side=Left
  wires:
  Demux/6 -> [Cm]
  [Cm] -> ThCA-/1
  [Cp] -> ThCA+/1
  [Bm] -> ThBC-/1
  [Bp] -> ThBC+/1
  [Am] -> ThAB-/1
  Demux/5 -> [Cp]
  Demux/4 -> [Bm]
  Demux/3 -> [Bp]
  Demux/2 -> [Am]
  Demux/1 -> [Ap]
  [Ap] -> ThAB+/1
  P/1 -> Demux/1
  connections:
  Lca/RConn1 -- Cca/LConn1
  Lbc/RConn1 -- Cbc/LConn1
  C/RConn1 -- ThCA+/LConn1 -- ThCA-/RConn1 -- Cbc/RConn1
  ThCA+/RConn1 -- ThCA-/LConn1 -- Lca/LConn1
  B/RConn1 -- ThBC+/LConn1 -- ThBC-/RConn1 -- Cab/RConn1
  ThBC+/RConn1 -- ThBC-/LConn1 -- Lbc/LConn1
  ThAB-/RConn1 -- ThAB+/LConn1 -- A/RConn1 -- Cca/RConn1
  ThAB+/RConn1 -- ThAB-/LConn1 -- Lab/LConn1
  Lab/RConn1 -- Cab/LConn1

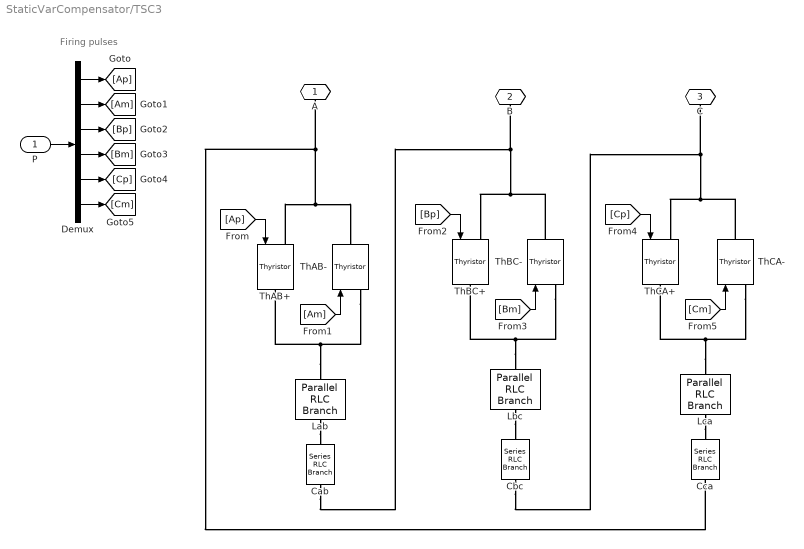
== system StaticVarCompensator/TSC3 ==
  note: Firing pulses
  P : Inport  PortDimensions=6
  Cab : spsSeriesRLCBranchLib/Series RLC Branch  LConnTagsString=__new0  RConnTagsString=__new0  BranchType=RC  Resistance=Rseries  Inductance=1.0  SetiL0=off  InitialCurrent=0  Capacitance=Ccmt  Setx0=off  InitialVoltage=0  Measurements=Branch voltage and current
  Cbc : spsSeriesRLCBranchLib/Series RLC Branch  LConnTagsString=__new0  RConnTagsString=__new0  BranchType=RC  Resistance=Rseries  Inductance=1.0  SetiL0=off  InitialCurrent=0  Capacitance=Ccmt  Setx0=off  InitialVoltage=0  Measurements=None
  Cca : spsSeriesRLCBranchLib/Series RLC Branch  LConnTagsString=__new0  RConnTagsString=__new0  BranchType=RC  Resistance=Rseries  Inductance=1.0  SetiL0=off  InitialCurrent=0  Capacitance=Ccmt  Setx0=off  InitialVoltage=0  Measurements=None
  Demux : Demux  Outputs=6
      settings: DisplayOption=none
  Lab : spsParallelRLCBranchLib/Parallel RLC Branch  LConnTagsString=a  RConnTagsString=__new0  BranchType=RL  Resistance=Rparallel  Inductance=Lcmt  SetiL0=off  InitialCurrent=0  Capacitance=1.0  Setx0=off  InitialVoltage=0  Measurements=None
  Lbc : spsParallelRLCBranchLib/Parallel RLC Branch  LConnTagsString=a  RConnTagsString=__new0  BranchType=RL  Resistance=Rparallel  Inductance=Lcmt  SetiL0=off  InitialCurrent=0  Capacitance=1.0  Setx0=off  InitialVoltage=0  Measurements=None
  Lca : spsParallelRLCBranchLib/Parallel RLC Branch  LConnTagsString=a  RConnTagsString=__new0  BranchType=RL  Resistance=Rparallel  Inductance=Lcmt  SetiL0=off  InitialCurrent=0  Capacitance=1.0  Setx0=off  InitialVoltage=0  Measurements=None
  ThAB+ : spsThyristorLib/Thyristor  Ron=Ron  Lon=0  Vf=Vf  IC=0  Rs=Rsnub  Cs=Csnub  Measurements=off
      settings: AttributesFormatString=\n
  ThAB- : spsThyristorLib/Thyristor  Ron=Ron  Lon=0  Vf=Vf  IC=0  Rs=inf  Cs=0  Measurements=off
      settings: AttributesFormatString=\n
  ThBC+ : spsThyristorLib/Thyristor  Ron=Ron  Lon=0  Vf=Vf  IC=0  Rs=Rsnub  Cs=Csnub  Measurements=off
      settings: AttributesFormatString=\n
  ThBC- : spsThyristorLib/Thyristor  Ron=Ron  Lon=0  Vf=Vf  IC=0  Rs=inf  Cs=0  Measurements=off
      settings: AttributesFormatString=\n
  ThCA+ : spsThyristorLib/Thyristor  Ron=Ron  Lon=0  Vf=Vf  IC=0  Rs=Rsnub  Cs=Csnub  Measurements=off
      settings: AttributesFormatString=\n
  ThCA- : spsThyristorLib/Thyristor  Ron=Ron  Lon=0  Vf=Vf  IC=0  Rs=inf  Cs=0  Measurements=off
      settings: AttributesFormatString=\n
  A : PMIOPort  Side=Left
  B : PMIOPort  Port=2  Side=Left
  C : PMIOPort  Port=3  Side=Left
  wires:
  P/1 -> Demux/1
  [Ap] -> ThAB+/1
  Demux/1 -> [Ap]
  Demux/2 -> [Am]
  Demux/3 -> [Bp]
  Demux/4 -> [Bm]
  Demux/5 -> [Cp]
  [Am] -> ThAB-/1
  [Bp] -> ThBC+/1
  [Bm] -> ThBC-/1
  [Cp] -> ThCA+/1
  [Cm] -> ThCA-/1
  Demux/6 -> [Cm]
  connections:
  Lab/RConn1 -- Cab/LConn1
  Lab/LConn1 -- ThAB-/LConn1 -- ThAB+/RConn1
  Cca/RConn1 -- A/RConn1 -- ThAB+/LConn1 -- ThAB-/RConn1
  Lbc/LConn1 -- ThBC-/LConn1 -- ThBC+/RConn1
  Cab/RConn1 -- ThBC-/RConn1 -- ThBC+/LConn1 -- B/RConn1
  Lca/LConn1 -- ThCA-/LConn1 -- ThCA+/RConn1
  Cbc/RConn1 -- ThCA-/RConn1 -- ThCA+/LConn1 -- C/RConn1
  Lbc/RConn1 -- Cbc/LConn1
  Lca/RConn1 -- Cca/LConn1

== system StaticVarCompensator/SVC Controller/3-phase signal generator ==
  Constant1 : Constant  Value=60
  Constant2 : Constant  Value=0.9998
  Constant3 : Constant  Value=-2
  Terminator : Terminator
  Three-Phase Sine Generator : spsThreePhaseSineGeneratorLib/Three-Phase Sine Generator  Ts=Ts
  abc : Outport  VectorParamsAs1DForOutWhenUnconnected=off
  wires:
  Constant1/1 -> Three-Phase Sine Generator/3
  Constant2/1 -> Three-Phase Sine Generator/1
  Constant3/1 -> Three-Phase Sine Generator/2
  Three-Phase Sine Generator/1 -> abc/1
  Three-Phase Sine Generator/2 -> Terminator/1

== system StaticVarCompensator/SVC Controller/Distribution Unit ==
  note: Bsec = ( 2 - Alpha/90 + sin(2*Alpha)/PI ) * Bsec_nom
  Bsvc : Inport  PortDimensions=1
  Bprim-->Bsec : Fcn  Expr=u[1]/(1 + u[1]*Xf_xfo*100e6/Pnom_xfo)
  Bsec --> Alpha : Lookup_n-D  NumberOfTableDimensions=1  BreakpointsForDimension1=B  BreakpointsForDimension2=[0 571.55 685.8 800.15 914.4 1028.8 1143.1 1257.4 1371.7 1486 1600.3 1714.6 1828.9 1943.2 2057.5 2171.8 2286.1 2400.5 2514.7 2629.1 2743.3 2857.7 2971.9 3086.3 3200.5 3314.9 3429.2]  Table=A  InternalRulePriority=Speed  RndMeth=Simplest
  Saturation : Saturate  UpperLimit=0  LowerLimit=Bpu_TCR
  Sum1 : Sum  Inputs=+---  InputSameDT=on  SaturateOnIntegerOverflow=on  OutDataTypeStr=Inherit: Same as first input
  TSC1 : Relay  OnSwitchValue=0  OffSwitchValue=-1 * hyst_svc
  TSC1+TSC2 : Relay  OnSwitchValue=0+ Bpu_TSC  OffSwitchValue=-1 * hyst_svc + Bpu_TSC
  TSC1+TSC2+TSC3 : Relay  OnSwitchValue=0+ 2*Bpu_TSC  OffSwitchValue=-1 * hyst_svc + 2*Bpu_TSC
  pu100_puLnom : Gain  Gain=-1/Bpu_TCR  SaturateOnIntegerOverflow=on  OutDataTypeStr=Inherit: Same as input  ParamDataTypeStr=Inherit: Same as input
  pu100_puLnom1 : Gain  Gain=Bpu_TSC  SaturateOnIntegerOverflow=on  OutDataTypeStr=Inherit: Same as input  ParamDataTypeStr=Inherit: Same as input
  pu100_puLnom2 : Gain  Gain=Bpu_TSC  SaturateOnIntegerOverflow=on  OutDataTypeStr=Inherit: Same as input  ParamDataTypeStr=Inherit: Same as input
  pu100_puLnom3 : Gain  Gain=Bpu_TSC  SaturateOnIntegerOverflow=on  OutDataTypeStr=Inherit: Same as input  ParamDataTypeStr=Inherit: Same as input
  Alpha : Outport  InitialOutput=0  VectorParamsAs1DForOutWhenUnconnected=off
  TSC1_On : Outport  Port=2  InitialOutput=0  VectorParamsAs1DForOutWhenUnconnected=off
  TSC2_On : Outport  Port=3  InitialOutput=0  VectorParamsAs1DForOutWhenUnconnected=off
  TSC3_On : Outport  Port=4  InitialOutput=0  VectorParamsAs1DForOutWhenUnconnected=off
  wires:
  pu100_puLnom/1 -> Bsec --> Alpha/1
  Bsec --> Alpha/1 -> Alpha/1
  Bsvc/1 -> Bprim-->Bsec/1
  Bprim-->Bsec/1 -> TSC1+TSC2+TSC3/1, TSC1+TSC2/1, TSC1/1, Sum1/1
  Saturation/1 -> pu100_puLnom/1
  Sum1/1 -> Saturation/1
  pu100_puLnom2/1 -> Sum1/3
  pu100_puLnom3/1 -> Sum1/2
  TSC1/1 -> TSC1_On/1, pu100_puLnom3/1
  TSC1+TSC2/1 -> TSC2_On/1, pu100_puLnom2/1
  pu100_puLnom1/1 -> Sum1/4
  TSC1+TSC2+TSC3/1 -> TSC3_On/1, pu100_puLnom1/1

== system StaticVarCompensator/SVC Controller/Firing Unit ==
  Vabc : Inport  PortDimensions=3
  Alpha : Inport  Port=2  PortDimensions=1
  TSC1_On : Inport  Port=3  PortDimensions=1
  TSC2_On : Inport  Port=4  PortDimensions=1
  TSC3_On : Inport  Port=5  PortDimensions=1
  Demux : Demux  Outputs=3
      settings: DisplayOption=none
  Firing Unit AB : Subsystem  mask{FiringMode=FiringMode, Nstep=Nstep, ParInit=[PhaseInit FreqInit], Ts=Ts}
      mask prompts: FiringMode "Firing Mode (1=Synchronized, 2=Continuous)"; Nstep "Total delay (in number of time step)"; ParInit "Initial phase and frequency of input: [ Phase (degree)  Freq (Hz) ]"; Ts "Sample time:"
      mask init:
      | PhaseInit=ParInit(1);
      | FreqInit=ParInit(2);
  Firing Unit BC : Subsystem  mask{FiringMode=FiringMode, Nstep=Nstep, ParInit=[PhaseInit-120  FreqInit], Ts=Ts}
      mask prompts: FiringMode "Firing Mode (1=Synchronized, 2=Continuous)"; Nstep "Total delay (in number of time step)"; ParInit "Initial phase and frequency of input: [ Phase (degree)  Freq (Hz) ]"; Ts "Sample time:"
      mask init:
      | PhaseInit=ParInit(1);
      | FreqInit=ParInit(2);
  Firing Unit CA : Subsystem  mask{FiringMode=FiringMode, Nstep=Nstep, ParInit=[PhaseInit+120  FreqInit], Ts=Ts}
      mask prompts: FiringMode "Firing Mode (1=Synchronized, 2=Continuous)"; Nstep "Total delay (in number of time step)"; ParInit "Initial phase and frequency of input: [ Phase (degree)  Freq (Hz) ]"; Ts "Sample time:"
      mask init:
      | PhaseInit=ParInit(1);
      | FreqInit=ParInit(2);
  Mux{,1..3} (4 alike) : Mux  Inputs=6
  V->pu : Gain  Gain=1/sqrt(3)  SaturateOnIntegerOverflow=on  OutDataTypeStr=Inherit: Same as input  ParamDataTypeStr=Inherit: Same as input
  TCR_Pulses : Outport  VectorParamsAs1DForOutWhenUnconnected=off
  TSC1_Pulses : Outport  Port=2  VectorParamsAs1DForOutWhenUnconnected=off
  TSC2_Pulses : Outport  Port=3  VectorParamsAs1DForOutWhenUnconnected=off
  TSC3_Pulses : Outport  Port=4  VectorParamsAs1DForOutWhenUnconnected=off
  wires:
  V->pu/1 -> Demux/1
  Alpha/1 -> Firing Unit AB/2(Alpha), Firing Unit CA/2(Alpha), Firing Unit BC/2(Alpha)
  TSC1_On/1 -> Firing Unit CA/3(TSC1_On), Firing Unit BC/3(TSC1_On), Firing Unit AB/3(TSC1_On)
  TSC2_On/1 -> Firing Unit CA/4(TSC2_On), Firing Unit BC/4(TSC2_On), Firing Unit AB/4(TSC2_On)
  Demux/1 -> Firing Unit AB/1(V)
  Demux/2 -> Firing Unit BC/1(V)
  Vabc/1 -> V->pu/1
  Demux/3 -> Firing Unit CA/1(V)
  Firing Unit AB/1(TCR +) -> Mux/1
  Firing Unit AB/2(TCR -) -> Mux/2
  Firing Unit BC/3(TSC1 +) -> Mux1/3
  Firing Unit BC/4(TSC1 -) -> Mux1/4
  Firing Unit BC/1(TCR +) -> Mux/3
  Firing Unit BC/2(TCR -) -> Mux/4
  Firing Unit CA/1(TCR +) -> Mux/5
  Firing Unit CA/2(TCR -) -> Mux/6
  Mux/1 -> TCR_Pulses/1
  Firing Unit AB/3(TSC1 +) -> Mux1/1
  Firing Unit AB/4(TSC1 -) -> Mux1/2
  Firing Unit CA/3(TSC1 +) -> Mux1/5
  Firing Unit CA/4(TSC1 -) -> Mux1/6
  Mux1/1 -> TSC1_Pulses/1
  Firing Unit AB/5(TSC2 +) -> Mux2/1
  Firing Unit AB/6(TSC2 -) -> Mux2/2
  Mux2/1 -> TSC2_Pulses/1
  Firing Unit BC/5(TSC2 +) -> Mux2/3
  Firing Unit BC/6(TSC2 -) -> Mux2/4
  Firing Unit CA/5(TSC2 +) -> Mux2/5
  Firing Unit CA/6(TSC2 -) -> Mux2/6
  TSC3_On/1 -> Firing Unit CA/5(TSC3_On), Firing Unit BC/5(TSC3_On), Firing Unit AB/5(TSC3_On)
  Mux3/1 -> TSC3_Pulses/1
  Firing Unit AB/7(TSC3 +) -> Mux3/1
  Firing Unit AB/8(TSC3 -) -> Mux3/2
  Firing Unit BC/7(TSC3 +) -> Mux3/3
  Firing Unit BC/8(TSC3 -) -> Mux3/4
  Firing Unit CA/7(TSC3 +) -> Mux3/5
  Firing Unit CA/8(TSC3 -) -> Mux3/6

== system StaticVarCompensator/SVC Controller/Info ==
  note: 1) Open-loop time constant evaluation:
  note: Xs -> Slope in pu/100MVA
      |  Ki -> Integral gain (puB/puV/s)
  note: where:
  note: Closed-loop time constant --> Tc ~= [ Xs / ( Xr + Xs ) ] * To
  note: Open-loop time constant --> To ~= 1 / ( Ki * Xs )
  note: To verify the following formula, open the loop (using the manual switch) and
      | add a 0.008 pu step to the reference voltage (Vref)
  note: 2) Misfiring simulation:
  note: To simulate a misfiring of thyristor AB+ of TSC1:
      | First switch off the TSC1 branch by adding a -0.008 pu to Vref at 0.04s
      | and then generate a firing pulse at 0.105s (one time step duration) using the Timer block

== system StaticVarCompensator/SVC Controller/Measurement System ==
  Vabc : Inport  PortDimensions=3
  PLL (3ph) : spsPLL3phLib/PLL (3ph)  Fmin=45  Par_Init=[Phase_Init Freq_Init]  ParK=[60 1400 0]  TcD=1e-4  MaxRateChangeFreq=12  FilterCutOffFreq=25  Ts=Ts  AGC=off
  Positive-Sequence (PLL-Driven) : spsPositiveSequencePLLDrivenLib/Positive-Sequence (PLL-Driven)  Finit=Freq_Init  Fmin=45  InInit=[Mag_Init 0]  Ts=Ts
  Terminator2 : Terminator
  Vmes : Outport  VectorParamsAs1DForOutWhenUnconnected=off
  wires:
  PLL (3ph)/1 -> Positive-Sequence (PLL-Driven)/1
  PLL (3ph)/2 -> Positive-Sequence (PLL-Driven)/2
  Vabc/1 -> Positive-Sequence (PLL-Driven)/3, PLL (3ph)/1
  Positive-Sequence (PLL-Driven)/2 -> Terminator2/1
  Positive-Sequence (PLL-Driven)/1 -> Vmes/1

== system StaticVarCompensator/SVC Controller/Voltage Regulator ==
  note: Xs -> Slope in pu/100MVA
      |  Ki -> Integral gain (puB/puV/s)
  note: where:
  note: Closed-loop time constant --> Tc = [ Xs / ( Xr + Xs ) ] * To
  note: Open-loop time constant --> To = 1 / ( Ki * Xs )
  Vmes : Inport  PortDimensions=1
  Bref : Inport  Port=2  PortDimensions=1
  Vref : Inport  Port=3
  Constant : Constant  Value=OpMode
  Constant10 : Constant
  Droop : Gain  Gain=Xs  SaturateOnIntegerOverflow=on  OutDataTypeStr=Inherit: Same as input  ParamDataTypeStr=Inherit: Same as input
  Gain1 : Gain  Gain=Kp  SaturateOnIntegerOverflow=on  OutDataTypeStr=Inherit: Same as input  ParamDataTypeStr=Inherit: Same as input
  Gain2 : Gain  Gain=Ki  SaturateOnIntegerOverflow=on  OutDataTypeStr=Inherit: Same as input  ParamDataTypeStr=Inherit: Same as input
  Integrateur : DiscreteIntegrator  SampleTime=Ts  LimitOutput=on  UpperSaturationLimit=Bmax  LowerSaturationLimit=Bmin  ICPrevOutput=DiscIntNeverNeededParam  ICPrevScaledInput=DiscIntNeverNeededParam
  Prod. : Product  InputSameDT=on  SaturateOnIntegerOverflow=on  OutDataTypeStr=Inherit: Same as first input
  Relational Operator2 : RelationalOperator  Operator=~=
  Som : Sum  Inputs=-+  InputSameDT=on  SaturateOnIntegerOverflow=on  OutDataTypeStr=Inherit: Same as first input
  Som1 : Sum  Inputs=-+  InputSameDT=on  SaturateOnIntegerOverflow=on  OutDataTypeStr=Inherit: Same as first input
  Som2 : Sum  InputSameDT=on  SaturateOnIntegerOverflow=on  OutDataTypeStr=Inherit: Same as first input
  Switch2 : Switch  Criteria=u2 > Threshold
  Unit Delay1 : UnitDelay  SampleTime=Ts  HasFrameUpgradeWarning=on
  Bsvc : Outport  InitialOutput=0  VectorParamsAs1DForOutWhenUnconnected=off
  wires:
  Constant/1 -> Relational Operator2/2
  Som1/1 -> Gain2/1, Gain1/1  "err"
  Gain2/1 -> Integrateur/1
  Relational Operator2/1 -> Switch2/2
  Bref/1 -> Switch2/1
  Som2/1 -> Switch2/3
  Switch2/1 -> Unit Delay1/1, Bsvc/1
  Vmes/1 -> Prod./1, Som/1
  Vref/1 -> Som/2
  Droop/1 -> Som1/1
  Som/1 -> Som1/2
  Constant10/1 -> Relational Operator2/1
  Unit Delay1/1 -> Prod./2
  Integrateur/1 -> Som2/2
  Gain1/1 -> Som2/1
  Prod./1 -> Droop/1
